simulink model "etc_no_bus"  (R2024a)
settings: Solver=VariableStepAuto  StartTime=0.0  StopTime=10.0  RelTol=1e-3  EnableMultiTasking=on
PreLoadFcn:
  | % Throttle body parameters
  | etc_plant_data;
values from neighbouring files (symbols this model uses):
  J = 0.000245    [allParamValues.mat]
  Kd = 0.03    [allParamValues.mat]
  Km = 3    [allParamValues.mat]
  Ks = 0.2    [allParamValues.mat]
  theta_eq = 0.523598775598    [allParamValues.mat]
libraries: simulink x1
settings Model: Creator=jrivitus  LastModifiedBy=bneiswan
settings SolverCC: AlgebraicLoopSolver=TrustRegion
settings DataIOCC: LimitDataPoints=on
settings OptimizationCC: ReuseModelBlockBuffer=off  ExpressionDepthLimit=2147483647  LifeSpan=inf
settings DebuggingCC: UnconnectedInputMsg=warning  UnconnectedOutputMsg=warning  UnconnectedLineMsg=warning  PregeneratedLibrarySubsystemCodeDiagnostic=none  SubsystemReferenceDiagnosticForUnitTest=warning
settings HardwareCC: ProdBitPerPointer=32  ProdBitPerSizeT=32  ProdBitPerPtrDiffT=32  ProdLargestAtomicFloat=None  ProdIntDivRoundTo=Undefined  ProdEndianess=Unspecified  ProdWordSize=32  ProdHWDeviceType=32-bit Generic
settings ModelReferenceCC: EnableRefExpFcnMdlSchedulingChecks=on  PropagateSignalLabelsOutOfModel=off
settings SFSimCC: SimUseLocalCustomCode=off
settings RTWCC: RTWUseLocalCustomCode=off  GPUComputeCapability=3.5  DLArmComputeVersion=19.05
settings CodeAppCC: StateflowObjectComments=on
settings GRTTargetCC: TargetLangStandard=C89/C90 (ANSI)  CombineOutputUpdateFcns=off  GRTInterface=on
settings ConfigComp: CovMetricSettings=dw  CovSaveCumulativeToWorkspaceVar=on  CovSaveSingleToWorkspaceVar=on  CovExternalEMLEnable=off  CovSFcnEnable=off

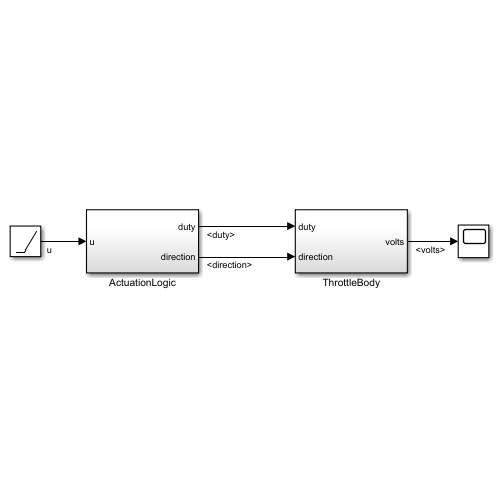
[thumbnail: Simulink's stored preview of the top-level diagram]
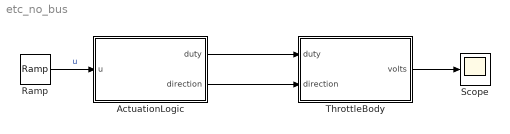
== system etc_no_bus ==
  ActuationLogic : Subsystem
  Ramp : simulink/Sources/Ramp  slope=0.4  start=0  InitialOutput=-2
  Scope : Scope
  ThrottleBody : Subsystem
  wires:
  Ramp/1 -> ActuationLogic/1(u)  "u"
  ThrottleBody/1(volts) -> Scope/1
  ActuationLogic/1(duty) -> ThrottleBody/1(duty)
  ActuationLogic/2(direction) -> ThrottleBody/2(direction)

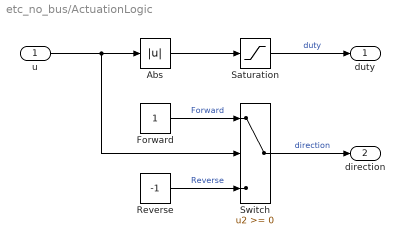
== system etc_no_bus/ActuationLogic ==
  u : Inport
  Abs : Abs  SaturateOnIntegerOverflow=off
  Forward : Constant  OutDataTypeStr=double
  Reverse : Constant  Value=-1  OutDataTypeStr=double
  Saturation : Saturate  UpperLimit=1  LowerLimit=0
      settings: AttributesFormatString=%<LowerLimit> < duty < %<UpperLimit>
  Switch : Switch  SaturateOnIntegerOverflow=off  InputSameDT=off
      settings: AttributesFormatString=Criteria: %<Criteria>\nThreshold: %<Threshold>
  duty : Outport
  direction : Outport  Port=2
  wires:
  Forward/1 -> Switch/1  "Forward"
  u/1 -> Abs/1, Switch/2
  Reverse/1 -> Switch/3  "Reverse"
  Saturation/1 -> duty/1  "duty"
  Switch/1 -> direction/1  "direction"
  Abs/1 -> Saturation/1

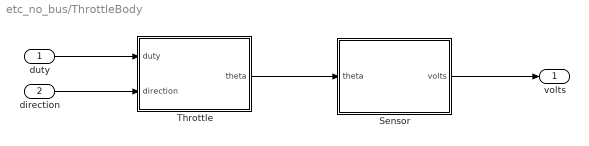
== system etc_no_bus/ThrottleBody ==
  duty : Inport
  direction : Inport  Port=2
  Sensor : Subsystem
  Throttle : Subsystem
  volts : Outport
  wires:
  Sensor/1(volts) -> volts/1
  Throttle/1(theta) -> Sensor/1(theta)
  duty/1 -> Throttle/1(duty)
  direction/1 -> Throttle/2(direction)

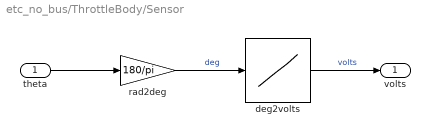
== system etc_no_bus/ThrottleBody/Sensor ==
  theta : Inport
  deg2volts : Lookup_n-D  NumberOfTableDimensions=1  BreakpointsForDimension1=[0 90]  Table=[0.5 4.5]  RndMeth=Simplest
  rad2deg : Gain  Gain=180/pi
  volts : Outport  VectorParamsAs1DForOutWhenUnconnected=off
  wires:
  rad2deg/1 -> deg2volts/1  "deg"
  deg2volts/1 -> volts/1  "volts"
  theta/1 -> rad2deg/1

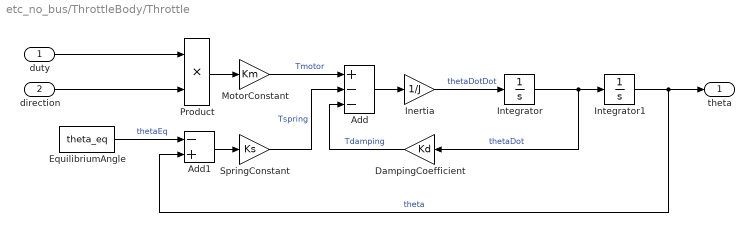
== system etc_no_bus/ThrottleBody/Throttle ==
  duty : Inport
  direction : Inport  Port=2
  Add : Sum  Inputs=+--
  Add1 : Sum  Inputs=-+
  DampingCoefficient : Gain  Gain=Kd
  EquilibriumAngle : Constant  Value=theta_eq
  Inertia : Gain  Gain=1/J
  Integrator : Integrator
      settings: AttributesFormatString=I.C. = %<InitialCondition>
  Integrator1 : Integrator  InitialCondition=theta_eq  LimitOutput=on  UpperSaturationLimit=pi/2  LowerSaturationLimit=0
      settings: AttributesFormatString=|
      | I.C. = %<InitialCondition>
      | %<LowerSaturationLimit><=theta<=%<UpperSaturationLimit>
  MotorConstant : Gain  Gain=Km
  Product : Product
  SpringConstant : Gain  Gain=Ks
  theta : Outport
  wires:
  DampingCoefficient/1 -> Add/3  "Tdamping"
  SpringConstant/1 -> Add/2  "Tspring"
  EquilibriumAngle/1 -> Add1/1  "thetaEq"
  Integrator/1 -> Integrator1/1, DampingCoefficient/1  "thetaDot"
  Integrator1/1 -> theta/1, Add1/2  "theta"
  Inertia/1 -> Integrator/1  "thetaDotDot"
  Product/1 -> MotorConstant/1
  Add1/1 -> SpringConstant/1
  Add/1 -> Inertia/1
  MotorConstant/1 -> Add/1  "Tmotor"
  duty/1 -> Product/1
  direction/1 -> Product/2
